simulink model "computedTorquePD"  (R2015a)
settings: Solver=ode3  StartTime=0.0  StopTime=10  RelTol=1e-3
libraries: simulink x4
settings Model: Creator=admin  LastModifiedBy=admin

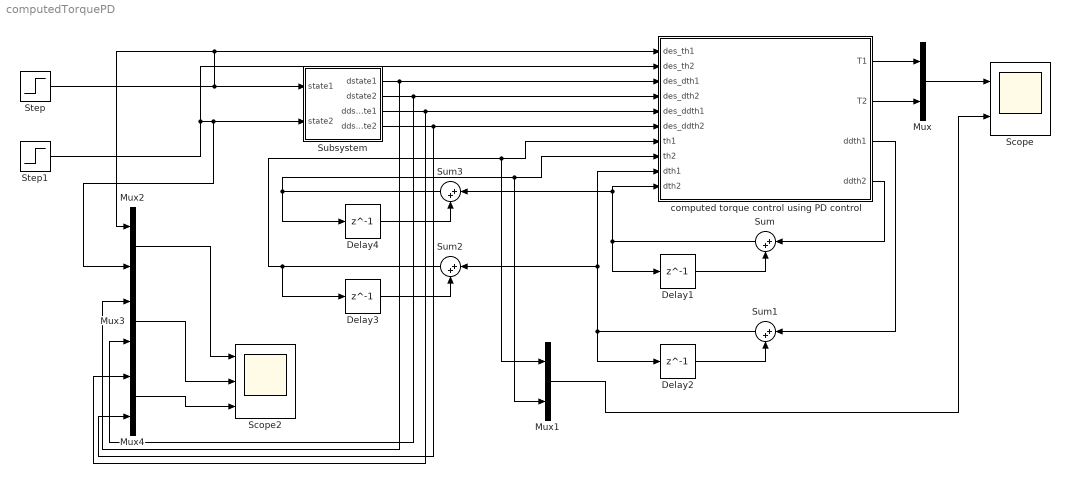
== system computedTorquePD ==
  Delay{1..4} (4 alike) : Delay  DelayLength=1  InitialCondition=0  SampleTime=1
  Mux{,1..4} (5 alike) : Mux  Inputs=2
  Scope : Scope  NumInputPorts=2
      settings: YMin=-5~-5  YMax=5~5
  Scope2 : Scope  NumInputPorts=3
      settings: YMin=-5~-5~-5  YMax=5~5~5  SaveName=ScopeData2
  Step : Step  Time=2  After=pi/3  SampleTime=0
  Step1 : Step  Time=0  After=0  SampleTime=0
  Subsystem : Subsystem
  Sum{,1..3} (4 alike) : Sum  Inputs=|++
  computed torque control using PD control : MATLAB Function  TreatAsAtomicUnit=on
  wires:
  Step1/1 -> computed torque control using PD control/2(des_th2), Mux2/2, Subsystem/2(state2)
  Sum2/1 -> Mux1/1, computed torque control using PD control/7(th1), Delay3/1
  computed torque control using PD control/4(ddth2) -> Sum/1
  Delay1/1 -> Sum/2
  computed torque control using PD control/3(ddth1) -> Sum1/1
  Delay2/1 -> Sum1/2
  Sum1/1 -> computed torque control using PD control/9(dth1), Sum2/1, Delay2/1
  Delay3/1 -> Sum2/2
  Sum3/1 -> Mux1/2, computed torque control using PD control/8(th2), Delay4/1
  Sum/1 -> Sum3/1, computed torque control using PD control/10(dth2), Delay1/1
  Delay4/1 -> Sum3/2
  Subsystem/1(dstate1) -> Mux3/1, computed torque control using PD control/3(des_dth1)
  Subsystem/2(dstate2) -> Mux3/2, computed torque control using PD control/4(des_dth2)
  Subsystem/3(ddstate1) -> Mux4/1, computed torque control using PD control/5(des_ddth1)
  Subsystem/4(ddstate2) -> computed torque control using PD control/6(des_ddth2), Mux4/2
  computed torque control using PD control/1(T1) -> Mux/1
  computed torque control using PD control/2(T2) -> Mux/2
  Mux/1 -> Scope/1
  Mux1/1 -> Scope/2
  Mux2/1 -> Scope2/1
  Mux3/1 -> Scope2/2
  Mux4/1 -> Scope2/3
  Step/1 -> computed torque control using PD control/1(des_th1), Mux2/1, Subsystem/1(state1)

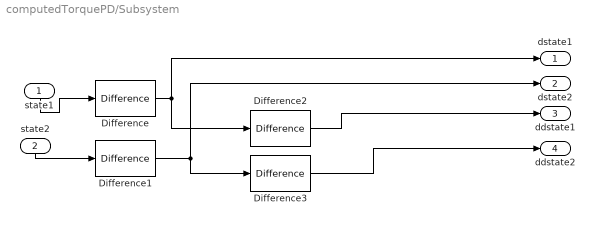
== system computedTorquePD/Subsystem ==
  state1 : Inport
  state2 : Inport  Port=2
  Difference{,1..3} (4 alike) : simulink/Discrete/Difference  ICPrevInput=0.0  InputProcessing=Inherited  OutMin=[]  OutMax=[]  OutDataType=fixdt(1, 16)  OutScaling=2^-10  DoSatur=off
  dstate1 : Outport
  dstate2 : Outport  Port=2
  ddstate1 : Outport  Port=3
  ddstate2 : Outport  Port=4
  wires:
  Difference2/1 -> ddstate1/1
  Difference3/1 -> ddstate2/1
  Difference/1 -> dstate1/1, Difference2/1
  state2/1 -> Difference1/1
  state1/1 -> Difference/1
  Difference1/1 -> dstate2/1, Difference3/1

== matlab function computedTorquePD/computed torque control using PD control ==
  data: des_th1 input; T1 output; des_th2 input; des_dth1 input; des_dth2 input; des_ddth1 input; des_ddth2 input; T2 output; ddth1 output; ddth2 output; th1 input; th2 input; dth1 input; dth2 input
function [T1,T2,ddth1,ddth2]    = fcn1(des_th1,des_th2,des_dth1,des_dth2,...
                                    des_ddth1,des_ddth2,th1,th2,...
                                    dth1,dth2)
%computed torque control method PD control
a1 = 0.20; a2 = 0.40; m1 = 2; m2 = 2; g = 9.8;
Kp = diag([0.1 0.1],0);
Kd = diag([1 1],0);             %for critical damping

h = 1;
des_dth1 = des_dth1/h;
des_dth2 = des_dth2/h;
des_ddth1 = des_ddth1/h;
des_ddth2 = des_ddth2/h;
dth1 = dth1/h;
dth2 = dth2/h;

T1 = 0;
T2 = 0;

D = [ ((a1^2*m1)/3 + a1^2*m2 + (a2^2*m2)/3)*ones + a1*a2*m2*cos(th2), (m2*a2^2)/3 + (a1*m2*cos(th2)*a2)/2;
                     (m2*a2^2)/3 + (a1*m2*cos(th2)*a2)/2,                            (a2^2*m2)/3];
H = [ -(a1*a2*m2*sin(th2)*(2*dth1 + dth2)*dth2)/2;
                                      (a1*a2*m2*sin(th2)*dth1^2)/2];
C = [ (a2*g*m2*cos(th1 + th2))/2 + (a1*g*m1*cos(th1))/2 + a1*g*m2*cos(th1);
                                                 (a2*g*m2*cos(th1 + th2))/2];
x = [th1; th2; dth1; dth2];
xdes = [des_th1; des_th2; des_dth1; des_dth2];
e = xdes-x;
u = -Kd*[e(3);e(4)]-Kp*[e(1);e(2)];
U = D*([des_ddth1;des_ddth2]-u)+H+C;
T1 = U(1);
T2 = U(2);
ddt = inv(D)*(U-H-C);
ddth1 = ddt(1);
ddth2 = ddt(2);
